simulink model "pfb_fir_16k_4tap_v3_core"  (Simulink 7.8)
settings: Solver=ode45  StartTime=0.0  StopTime=10.0  RelTol=1e-3
libraries: xbsIndex_r4 x287, casper_library_misc x8
(part 2 of 9)

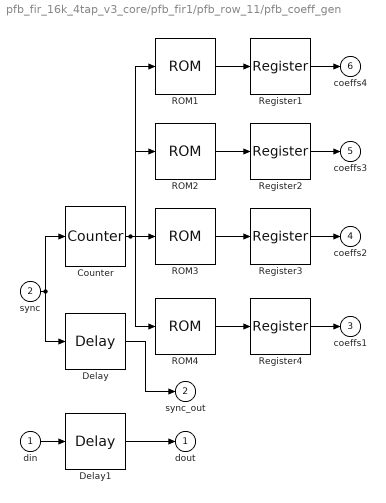
== system pfb_fir_16k_4tap_v3_core/pfb_fir1/pfb_row_11/pfb_coeff_gen ==
  din : Inport
  sync : Inport  Port=2
  Counter : xbsIndex_r4/Counter  cnt_type=Free Running  cnt_to=Inf  operation=Up  start_count=0  cnt_by_val=1  arith_type=Unsigned  n_bits=12  bin_pt=0  load_pin=off  rst=on  en=off  explicit_period=on  period=1  dbl_ovrd=off  use_behavioral_HDL=off  implementation=Fabric  use_rpm=on  block_type=counter
  Delay : xbsIndex_r4/Delay  rst=off  infoeditControl=Selection of Reset will increase slice count due to use of real FFs and instead of SRLs  en=off  latency=4  dbl_ovrd=off  reg_retiming=off  block_type=delay
  Delay1 : xbsIndex_r4/Delay  rst=off  infoeditControl=Selection of Reset will increase slice count due to use of real FFs and instead of SRLs  en=off  latency=4  dbl_ovrd=off  reg_retiming=off  block_type=delay
  ROM1 : xbsIndex_r4/ROM  depth=4096  initVector=[-3.1185374660155e-18 -9.76682041058843e-06 -1.95360449163731e-05 -2.93076934355949e-05 -3.90817858961647e-05 -4.88583422355305e-05 -5.86373824007115e-05 -6.84189263482179e-05 -7.82029940439724e-05 -8.7989605463343e-05 -9.77787805910074e-05 -0.000107570539420998 -0.000117364901956564 -0.000127161888210209 -0.000136961518203607 -0.000146763811967525 -0.000156568789541854 -0.000166376470975477 -0.000176186876326299 -0.000186000025661167 -0.000195815939055794 -0.000205634636594785 -0.000215456138371508 -0.000225280464488124 -0.000235107635055507 -0.000244937670193162 -0.000254770590029263 -0.000264606414700512 -0.000274445164352173 -0.000284286859137995 -0.000294131519220126 -0.000303979164769151 -0.000313829815963953 -0.000323683492991758 -0.000333540216047996 -0.000343400005336337 -0.000353262881068609 -0.000363128863464718 -0.000372997972752678 -0.000382870229168479 -0.000392745652956117 -0.000402624264367512 -0.000412506083662428 -0.000422391131108511 -0.000432279426981142 -0.000442170991563478 -0.000452065845146367 -0.000461964008028269 -0.000471865500515287 -0.000481770342921032 -0.000491678555566652 -0.000501590158780754 -0.000511505172899322 -0.000521423618265749 -0.0005313455152307 -0.000541270884152156 -0.000551199745395276 -0.000561132119332427 -0.000571068026343107 -0.000581007486813861 -0.000590950521138314 -0.000600897149717034 -0.000610847392957561 -0.00062080127127433 -0.000630758805088587 -0.000640720014828422 -0.00065068492092863 -0.000660653543830745 -0.000670625903982955 -0.000680602021840026 -0.000690581917863328 -0.0007005656125207 -0.000710553126286484 -0.000720544479641437 -0.000730539693072656 -0.000740538787073605 -0.000750541782143982 -0.000760548698789756 -0.000770559557523031 -0.000780574378862079 -0.000790593183331257 -0.000800615991460928 -0.000810642823787486 -0.000820673700853222 -0.000830708643206358 -0.000840747671400958 -0.000850790805996856 -0.000860838067559675 -0.000870889476660698 -0.000880945053876898 -0.00089100481979085 -0.000901068794990657 -0.000911137000069975 -0.000921209455627878 -0.000931286182268886 -0.000941367200602888 -0.000951452531245053 -0.000961542194815867 -0.000971636211940989 -0.000981734603251297 -0.000991837389382751 -0.00100194459097642 -0.00101205622867839 -0.00102217232313971 -0.0010322928950164 -0.00104241796496931 -0.00105254755366415 -0.00106268168177145 -0.0010728203699664 -0.00108296363892896 -0.00109311150934365 -0.00110326400189965 -0.00111342113729066 -0.00112358293621484 -0.00113374941937486 -0.00114392060747772 -0.00115409652123481 -0.00116427718136181 -0.00117446260857864 -0.00118465282360944 -0.00119484784718247 -0.00120504770003014 -0.00121525240288887 -0.00122546197649911 -0.00123567644160527 -0.00124589581895565 -0.00125612012930244 -0.00126634939340158 -0.00127658363201284 -0.00128682286589967 -0.00129706711582917 -0.00130731640257208 -0.00131757074690268 -0.00132783016959879 -0.00133809469144168 -0.00134836433321602 -0.0013586391157099 -0.00136891905971467 -0.00137920418602497 -0.0013894945154387 -0.00139979006875685 -0.00141009086678361 -0.00142039693032617 -0.00143070828019481 -0.00144102493720273 -0.00145134692216608 -0.00146167425590389 -0.00147200695923797 -0.00148234505299297 -0.0014926885579962 -0.00150303749507769 -0.00151339188507009 -0.00152375174880858 -0.00153411710713095 -0.00154448798087738 -0.00155486439089054 -0.00156524635801545 -0.00157563390309945 -0.00158602704699218 -0.00159642581054548 -0.00160683021461339 -0.00161724028005209 -0.00162765602771979 -0.00163807747847678 -0.00164850465318529 -0.0016589375727095 -0.00166937625791546 -0.00167982072967105 -0.00169027100884594 -0.00170072711631149 -0.0017111890729408 -0.00172165689960852 -0.00173213061719096 -0.0017426102465659 -0.00175309580861261 -0.00176358732421181 -0.00177408481424555 -0.00178458829959727 -0.00179509780115164 -0.00180561333979455 -0.00181613493641312 -0.00182666261189554 -0.00183719638713109 -0.0018477362830101 -0.00185828232042384 -0.00186883452026453 ...(+78457 chars)]  distributed_mem=Block RAM  rst=off  init_reg=0  en=off  latency=3  gui_display_data_type=Fixed-point  arith_type="Signed  (2's comp)"  n_bits=18  bin_pt=17  preci_type=Single  exp_width=8  frac_width=24  dbl_ovrd=off  optimize=Area  use_rpm=on  block_type=sprom
  ROM2 : xbsIndex_r4/ROM  depth=4096  initVector=[2.1050557694588e-17 0.000131913890883874 0.000263978326654002 0.000396193339848099 0.000528558962909183 0.000661075228185063 0.000793742167928575 0.000926559814297439 0.00105952819935419 0.00119264735506601 0.00132591731330502 0.00145933810584769 0.0015929097643751 0.0017266323204728 0.00186050580563066 0.0019945302512431 0.00212870568860859 0.00226303214892984 0.00239750966331368 0.002532138262771 0.0026669179782166 0.00280184884046941 0.00293693088025198 0.0030721641281907 0.0032075486148157 0.00334308437056062 0.00347877142576296 0.00361460981066343 0.00375059955540629 0.00388674069003916 0.00402303324451295 0.0041594772486817 0.00429607273230289 0.00443281972503683 0.00456971825644691 0.00470676835599953 0.00484397005306387 0.00498132337691215 0.00511882835671914 0.00525648502156236 0.00539429340042195 0.00553225352218061 0.00567036541562341 0.00580862910943813 0.0059470446322146 0.00608561201244507 0.00622433127852396 0.00636320245874778 0.00650222558131537 0.0066414006743273 0.00678072776578623 0.00692020688359665 0.00705983805556488 0.00719962130939893 0.0073395566727087 0.00747964417300547 0.00761988383770216 0.00776027569411317 0.00790081976945423 0.00804151609084266 0.00818236468529683 0.0083233655797364 0.00846451880098218 0.00860582437575608 0.00874728233068094 0.00888889269228079 0.00903065548698031 0.0091725707411051 0.00931463848088149 0.00945685873243645 0.00959923152179779 0.00974175687489367 0.00988443481755281 0.0100272653755043 0.0101702485743778 0.0103133844397029 0.01045667299691 0.010600114271329 0.0107437082881904 0.0108874550726246 0.0110313546496618 0.0111754070442324 0.0113196122811666 0.0114639703851941 0.0116084813809446 0.0117531452929474 0.0118979621456312 0.0120429319633247 0.0121880547702556 0.0123333305905512 0.012478759448238 0.0126243413672418 0.0127700763713879 0.0129159644844004 0.0130620057299026 0.0132082001314168 0.0133545477123643 0.0135010484960652 0.0136477025057385 0.0137945097645021 0.0139414702953722 0.0140885841212641 0.0142358512649913 0.0143832717492661 0.014530845596699 0.0146785728297992 0.0148264534709739 0.0149744875425286 0.0151226750666672 0.0152710160654918 0.0154195105610021 0.0155681585750963 0.0157169601295704 0.015865915246118 0.016015023946331 0.0161642862516988 0.0163137021836086 0.016463271763345 0.0166129950120905 0.0167628719509248 0.0169129026008255 0.0170630869826672 0.0172134251172219 0.0173639170251589 0.0175145627270447 0.0176653622433432 0.017816315594415 0.0179674228005178 0.0181186838818066 0.0182700988583328 0.018421667750045 0.0185733905767885 0.0187252673583054 0.0188772981142341 0.0190294828641101 0.0191818216273651 0.0193343144233273 0.0194869612712216 0.019639762190169 0.0197927171991867 0.0199458263171884 0.0200990895629838 0.0202525069552789 0.0204060785126757 0.020559804253672 0.0207136841966617 0.0208677183599346 0.0210219067616763 0.0211762494199682 0.0213307463527873 0.0214853975780062 0.0216402031133933 0.0217951629766123 0.0219502771852226 0.0221055457566788 0.0222609687083309 0.0224165460574242 0.0225722778210991 0.0227281640163916 0.0228842046602324 0.0230403997694473 0.0231967493607572 0.0233532534507779 0.02350991205602 0.0236667251928893 0.0238236928776857 0.0239808151266045 0.024138091955735 0.0242955233810616 0.024453109418463 0.0246108500837125 0.0247687453924776 0.0249267953603203 0.025085000002697 0.025243359334958 0.0254018733723483 0.0255605421300066 0.0257193656229659 0.025878343866153 0.0260374768743888 0.0261967646623882 0.0263562072447599 0.0265158046360062 0.0266755568505233 0.026835463902601 0.0269955258064227 0.0271557425760656 0.0273161142255001 0.0274766407685902 0.0276373222190932 0.0277981585906598 0.0279591498968342 0.0281202961510533 0.0282815973666477 0.0284430535568408 0.0286046647347492 0.0287664309133822 0.0289283521056427 0.0290904283243259 0.0292526595821201 0.0294150458916062 0.0295775872652578 0.0297402837154417 0.0299031352544167 0.0300661418943344 0.0302293036472389 0.0303926205250668 0.0305560925396469 ...(+69912 chars)]  distributed_mem=Block RAM  rst=off  init_reg=0  en=off  latency=3  gui_display_data_type=Fixed-point  arith_type="Signed  (2's comp)"  n_bits=18  bin_pt=17  preci_type=Single  exp_width=8  frac_width=24  dbl_ovrd=off  optimize=Area  use_rpm=on  block_type=sprom
  ROM3 : xbsIndex_r4/ROM  depth=4096  initVector=[0.999999999471456 0.99999985914225 0.999999455068117 0.9999987872493 0.999997855686203 0.999996660379388 0.999995201329576 0.999993478537646 0.999991492004636 0.999989241731742 0.999986727720322 0.999983949971888 0.999980908488115 0.999977603270834 0.999974034322036 0.999970201643871 0.999966105238646 0.999961745108828 0.999957121257044 0.999952233686077 0.999947082398871 0.999941667398528 0.999935988688307 0.99993004627163 0.999923840152073 0.999917370333374 0.999910636819428 0.999903639614289 0.999896378722171 0.999888854147444 0.99988106589464 0.999873013968448 0.999864698373715 0.999856119115448 0.999847276198812 0.999838169629131 0.999828799411888 0.999819165552723 0.999809268057437 0.999799106931989 0.999788682182496 0.999777993815232 0.999767041836634 0.999755826253295 0.999744347071966 0.999732604299557 0.999720597943139 0.999708328009939 0.999695794507343 0.999682997442896 0.999669936824303 0.999656612659424 0.999643024956282 0.999629173723055 0.999615058968082 0.999600680699859 0.999586038927041 0.999571133658442 0.999555964903035 0.99954053266995 0.999524836968477 0.999508877808063 0.999492655198315 0.999476169148999 0.999459419670036 0.999442406771511 0.999425130463662 0.999407590756889 0.999389787661749 0.999371721188959 0.999353391349393 0.999334798154083 0.99931594161422 0.999296821741156 0.999277438546396 0.999257792041609 0.999237882238619 0.999217709149409 0.999197272786121 0.999176573161056 0.999155610286672 0.999134384175584 0.99911289484057 0.999091142294562 0.999069126550651 0.999046847622089 0.999024305522283 0.999001500264801 0.998978431863367 0.998955100331864 0.998931505684334 0.998907647934978 0.998883527098152 0.998859143188374 0.998834496220317 0.998809586208814 0.998784413168856 0.998758977115593 0.99873327806433 0.998707316030534 0.998681091029828 0.998654603077994 0.998627852190971 0.998600838384857 0.998573561675908 0.998546022080538 0.998518219615319 0.99849015429698 0.998461826142411 0.998433235168656 0.998404381392921 0.998375264832567 0.998345885505114 0.998316243428241 0.998286338619783 0.998256171097734 0.998225740880246 0.998195047985628 0.998164092432349 0.998132874239034 0.998101393424466 0.998069650007586 0.998037644007493 0.998005375443444 0.997972844334854 0.997940050701295 0.997906994562497 0.997873675938348 0.997840094848894 0.997806251314338 0.99777214535504 0.99773777699152 0.997703146244454 0.997668253134677 0.997633097683178 0.997597679911109 0.997561999839776 0.997526057490642 0.997489852885331 0.997453386045621 0.99741665699345 0.997379665750912 0.99734241234026 0.997304896783902 0.997267119104406 0.997229079324496 0.997190777467054 0.99715221355512 0.997113387611889 0.997074299660715 0.997034949725111 0.996995337828743 0.99695546399544 0.996915328249183 0.996874930614112 0.996834271114527 0.996793349774881 0.996752166619787 0.996710721674013 0.996669014962487 0.996627046510292 0.996584816342669 0.996542324485015 0.996499570962885 0.996456555801991 0.996413279028203 0.996369740667546 0.996325940746203 0.996281879290514 0.996237556326976 0.996192971882243 0.996148125983125 0.996103018656591 0.996057649929764 0.996012019829927 0.995966128384516 0.995919975621127 0.995873561567512 0.99582688625158 0.995779949701395 0.995732751945179 0.995685293011311 0.995637572928326 0.995589591724916 0.99554134942993 0.995492846072372 0.995444081681404 0.995395056286345 0.995345769916669 0.995296222602007 0.995246414372147 0.995196345257033 0.995146015286766 0.995095424491601 0.995044572901954 0.994993460548393 0.994942087461644 0.99489045367259 0.994838559212269 0.994786404111876 0.994733988402761 0.994681312116432 0.994628375284553 0.994575177938942 0.994521720111576 0.994468001834586 0.994414023140259 0.99435978406104 0.994305284629528 0.99425052487848 0.994195504840806 0.994140224549575 0.99408468403801 0.99402888333949 0.993972822487551 0.993916501515884 0.993859920458336 0.993803079348909 0.993745978221762 0.993688617111209 0.99363099605172 0.99357311507792 0.99351497422459 ...(+69915 chars)]  distributed_mem=Block RAM  rst=off  init_reg=0  en=off  latency=3  gui_display_data_type=Fixed-point  arith_type="Signed  (2's comp)"  n_bits=18  bin_pt=17  preci_type=Single  exp_width=8  frac_width=24  dbl_ovrd=off  optimize=Area  use_rpm=on  block_type=sprom
  ROM4 : xbsIndex_r4/ROM  depth=4096  initVector=[2.10488384986554e-17 -0.000131752614018843 -0.000263354753776292 -0.000394806452101551 -0.000526107741918696 -0.000657258656246122 -0.000788259228196784 -0.000919109490978046 -0.00104980947789161 -0.00118035922233338 -0.00131075875779367 -0.00144100811785671 -0.00157110733620086 -0.00170105644659846 -0.0018308554829157 -0.00196050447911283 -0.00209000346924366 -0.00221935248745577 -0.00234855156799037 -0.00247760074518224 -0.00260650005345958 -0.0027352495273442 -0.00286384920145108 -0.0029922991104885 -0.00312059928925799 -0.00324874977265411 -0.00337675059566472 -0.00350460179337042 -0.00363230340094483 -0.00375985545365441 -0.00388725798685839 -0.00401451103600861 -0.0041416146366498 -0.00426856882441899 -0.00439537363504579 -0.00452202910435222 -0.00464853526825256 -0.00477489216275358 -0.00490109982395405 -0.0050271582880449 -0.00515306759130914 -0.00527882777012174 -0.00540443886094953 -0.00552990090035136 -0.00565521392497764 -0.00578037797157053 -0.00590539307696383 -0.00603025927808279 -0.00615497661194434 -0.0062795451156566 -0.00640396482641909 -0.00652823578152257 -0.00665235801834898 -0.0067763315743713 -0.00690015648715373 -0.00702383279435124 -0.00714736053370974 -0.00727073974306595 -0.00739397046034725 -0.00751705272357192 -0.00763998657084858 -0.00776277204037646 -0.00788540917044522 -0.00800789799943488 -0.0081302385658157 -0.00825243090814835 -0.00837447506508347 -0.00849637107536178 -0.00861811897781405 -0.00873971881136088 -0.00886117061501292 -0.00898247442787039 -0.00910363028912329 -0.00922463823805123 -0.00934549831402337 -0.00946621055649828 -0.00958677500502412 -0.0097071916992382 -0.00982746067886712 -0.00994758198372667 -0.0100675556537217 -0.0101873817288462 -0.0103070602491829 -0.0104265912549037 -0.0105459747862691 -0.0106652108836283 -0.0107842995874191 -0.0109032409381682 -0.0110220349764904 -0.0111406817430893 -0.0112591812787565 -0.011377533624372 -0.0114957388209041 -0.0116137969094092 -0.0117317079310315 -0.0118494719270034 -0.0119670889386453 -0.012084559007365 -0.0122018821746584 -0.0123190584821091 -0.012436087971388 -0.0125529706842538 -0.0126697066625522 -0.0127862959482169 -0.0129027385832683 -0.0130190346098144 -0.0131351840700501 -0.0132511870062574 -0.0133670434608053 -0.0134827534761498 -0.0135983170948335 -0.0137137343594861 -0.0138290053128234 -0.0139441299976484 -0.0140591084568502 -0.0141739407334047 -0.0142886268703737 -0.0144031669109057 -0.0145175608982352 -0.0146318088756827 -0.0147459108866552 -0.0148598669746453 -0.0149736771832316 -0.0150873415560785 -0.015200860136936 -0.0153142329696403 -0.0154274600981125 -0.0155405415663596 -0.0156534774184741 -0.0157662676986335 -0.0158789124511009 -0.0159914117202244 -0.0161037655504375 -0.0162159739862584 -0.0163280370722904 -0.0164399548532217 -0.0165517273738254 -0.0166633546789591 -0.0167748368135654 -0.016886173822671 -0.0169973657513876 -0.0171084126449108 -0.0172193145485211 -0.0173300715075829 -0.0174406835675447 -0.0175511507739394 -0.0176614731723836 -0.0177716508085783 -0.0178816837283079 -0.0179915719774408 -0.0181013156019291 -0.0182109146478085 -0.0183203691611982 -0.018429679188301 -0.018538844775403 -0.0186478659688737 -0.0187567428151656 -0.0188654753608147 -0.0189740636524398 -0.0190825077367428 -0.0191908076605085 -0.0192989634706046 -0.0194069752139815 -0.019514842937672 -0.0196225666887922 -0.01973014651454 -0.0198375824621961 -0.0199448745791234 -0.0200520229127673 -0.0201590275106552 -0.0202658884203966 -0.0203726056896832 -0.0204791793662886 -0.0205856094980681 -0.020691896132959 -0.0207980393189804 -0.0209040391042327 -0.0210098955368982 -0.0211156086652404 -0.0212211785376044 -0.0213266052024165 -0.0214318887081843 -0.0215370291034965 -0.021642026437023 -0.0217468807575144 -0.0218515921138025 -0.0219561605547998 -0.0220605861294997 -0.0221648688869761 -0.0222690088763834 -0.0223730061469568 -0.0224768607480117 -0.0225805727289439 -0.0226841421392295 -0.0227875690284249 -0.0228908534461662 ...(+78449 chars)]  distributed_mem=Block RAM  rst=off  init_reg=0  en=off  latency=3  gui_display_data_type=Fixed-point  arith_type="Signed  (2's comp)"  n_bits=18  bin_pt=17  preci_type=Single  exp_width=8  frac_width=24  dbl_ovrd=off  optimize=Area  use_rpm=on  block_type=sprom
  Register{1..4} (4 alike) : xbsIndex_r4/Register  init=0  rst=off  en=off  dbl_ovrd=off  block_type=register
  dout : Outport
  sync_out : Outport  Port=2
  coeffs1 : Outport  Port=3
  coeffs2 : Outport  Port=4
  coeffs3 : Outport  Port=5
  coeffs4 : Outport  Port=6
  wires:
  sync/1 -> Delay/1, Counter/1
  Counter/1 -> ROM1/1, ROM2/1, ROM3/1, ROM4/1
  Register1/1 -> coeffs4/1
  ROM1/1 -> Register1/1
  Register2/1 -> coeffs3/1
  ROM2/1 -> Register2/1
  Register3/1 -> coeffs2/1
  ROM3/1 -> Register3/1
  Register4/1 -> coeffs1/1
  ROM4/1 -> Register4/1
  Delay1/1 -> dout/1
  din/1 -> Delay1/1
  Delay/1 -> sync_out/1
